simulink model "step3c"  (Simulink 8.5)
settings: Solver=ode15s  SolverMode=SingleTasking  StartTime=0.0  StopTime=0.199  RelTol=1e-4  AbsTol=1e-6
undefined symbols (not defined in the file or in its folder): den, dx, num
libraries: elements x1
settings Model: Creator=PC  LastModifiedBy=PC
settings DataIOCC: LimitDataPoints=off
settings OptimizationCC: BlockReduction=off  BooleanDataType=off  ExpressionDepthLimit=128
settings DebuggingCC: SaveWithParameterizedLinksMsg=none  SignalResolutionControl=TryResolveAllWithWarning  MultiTaskDSMMsg=warning  MultiTaskCondExecSysMsg=none  FcnCallInpInsideContextMsg=EnableAllAsError  StateNameClashWarn=none  StrictBusMsg=None
settings HardwareCC: TargetUnknown=on
settings RTWCC: TemplateMakefile=grt_vc.tmf

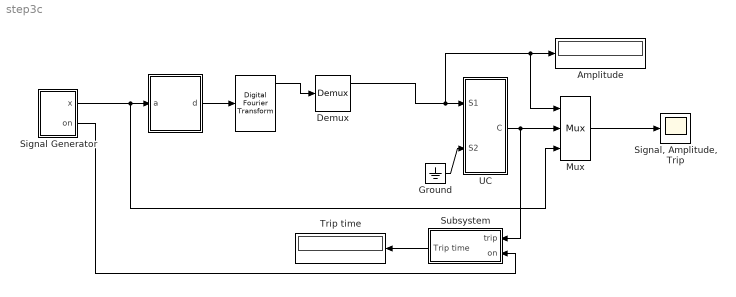
== system step3c ==
  " " : elements/   fo=60  window_size=20  harmonic=[1 2 3 4 5]
  "  " : Subsystem  mask(Data Adquisition Board){filter=on, approx=Butterworth, order=3, numerator=[], denominator=[], freq=180, resdis=on, vertres=8, xmax=100, winsize=20, G=1.0, fs=60*20}
      mask prompts: filter "Disable Analog Filter"; approx "Filter approximation"; numerator "Free expression filter: numerator(descending order of s)"; denominator "Free expression filter: denominator:"; freq "Cut-off frequency"; resdis "Disable Vertical Resolution"; vertres "Vertical Resolution: No. of bits"; xmax "Vertical Resolution: signal range"; winsize "Window size"; G "Gain"; fs "Sampling frequency"
      mask help: Takes the instantaneous value of the input signal and convert it to the data window of samples.
      mask init:
      | dab1
      mask TypeOptions approx: Bessel | Tschebyscheff | Butterworth | free expression
      mask TypeOptions order: 2 | 3 | 4
      mask TypeOptions vertres: 8 | 12 | 16
      mask Display: disp('DAB')
  Amplitude : Display
  Demux : Demux  Outputs=2
  Ground : Ground
  Mux : Mux  Inputs=3
  Signal Generator : Subsystem  mask(Signal Generator){A1=2, f1=60, A2=0, f2=2*60, A3=0, f3=1500, tstart=1.25/60}
      mask prompts: A1 "Amplitude 1"; f1 "Frequency 1 [Hz]"; A2 "Amplitude 2"; f2 "Frequency 2 [Hz]"; A3 "Amplitude 3"; f3 "Frequency 3 [Hz]"; tstart "Start time [sec]"
  "Signal, Amplitude, Trip" : Scope
      settings: TickLabels=on  YMin=-4.5  YMax=4.5
  Subsystem : Subsystem
  Trip time : Display
  UC : Subsystem  mask(Universal Comparator){type2=Signal-Time, sign=>, Ipickup=0.75, k1=0.95, type1=Very Inverse, type3=Present value, k=0.015, fs=20*60}
      mask prompts: type2 "Type of comparison"; Ipickup "Pick-up value:"; k1 "Ratio of reset to pick-up:"; type1 "Type of Time dependency"; type3 "I-t emulation method"; k "Time parameter (seconds):"; fs "Sampling frecuency (Hz):"
      mask help: This block is an Universal Comparator. It can perform a comparison between a signal an a threshold or two signals. It can also emulate some time-signal characteristics.
      mask init:
      | switch type2,
      |    case 1,
      |        %signal-threshold
      |        if sign ==1
      |           %S1>S2
      |           aux=0;
      |        else
      |           %S1<S2
      |           aux=1;
      |        end;
      |    case 2,
      |        %Signal-Signal
      |       if sign ==1
      |           aux=2;
      |    	else
      |          aux=3;
      |       end;
      |    case 3,
      |       %signal-time
      |       if type3==1
      |          %instantaneous value of input signal
      |          switch type1,
      |             case 1,
      |                %time defined
      |                aux=4;
      |             case 2,
      |                %inverse time
      |                aux=6;
      |             case 3,
      |                %very inverse
      |                aux=7;
      |             case 4,
      |                %extremely inverse
      |                aux=8;
      |             case 5,
      |                %RI inverse
      |                aux=9;
      |             case 6,
      |                %Long time inverse
      |                aux=10;
      |             otherwise,
      |                aux=0;
      |          end;
      |       else
      |          switch type1,
      |             case 1,
      |                %time defined
      |                aux=5;
      |             case 2,
      |                %inverse time
      |                aux=11;
      |             case 3,
      |                %very inverse
      |                aux=12;
      |             case 4,
      |                %extremely inverse
      |                aux=13;
      |             case 5,
      |                %RI inverse
      |                aux=14;
      |             case 6,
      |                %Long time inverse
      |                aux=15;
      |             otherwise,
      |                aux=0;
      |          end;
      |       end;
      |    otherwise,
      |          aux=0;
      | end;
      mask TypeOptions type2: Signal-Threshold | Signal-Signal | Signal-Time
      mask TypeOptions sign: > | <
      mask TypeOptions type1: Time defined | Standard Inverse | Very Inverse | Extra Inverse | RI Inverse | Long Time Inverse
      mask TypeOptions type3: Present value | integration
      mask Display: disp('UC');
  wires:
  Signal Generator/1(x) -> "  "/1(a), Mux/3
  "  "/1(d) -> " "/1
  " "/1 -> Demux/1
  Signal Generator/2(on) -> Subsystem/2(on)
  Subsystem/1(Trip time) -> Trip time/1
  UC/1(C) -> Subsystem/1(trip), Mux/2
  Mux/1 -> "Signal, Amplitude, Trip"/1
  Ground/1 -> UC/2(S2)
  Demux/1 -> UC/1(S1), Amplitude/1, Mux/1

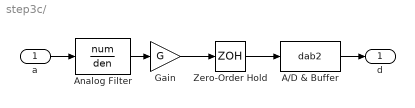
== system step3c/   ==
  a : Inport
  A/D & Buffer : S-Function  FunctionName=dab2  Parameters=winsize,fs,dx,resdis
  Analog Filter : TransferFcn  Numerator=num  Denominator=den
  Gain : Gain  Gain=G  SaturateOnIntegerOverflow=on  OutDataTypeStr=Inherit: Same as input  ParamDataTypeStr=Inherit: Same as input
  Zero-Order Hold : ZeroOrderHold  SampleTime=1/fs
  d : Outport  InitialOutput=[zeros(winsize,1)]
  wires:
  A/D & Buffer/1 -> d/1
  a/1 -> Analog Filter/1
  Zero-Order Hold/1 -> A/D & Buffer/1
  Gain/1 -> Zero-Order Hold/1
  Analog Filter/1 -> Gain/1

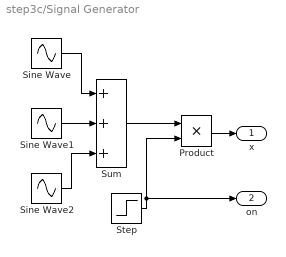
== system step3c/Signal Generator ==
  Product : Product  SaturateOnIntegerOverflow=on  RndMeth=Zero  InputSameDT=on  OutDataTypeStr=Inherit: Same as first input
  Sine Wave : Sin  Amplitude=A1  Frequency=f1*2*pi  SampleTime=0
  Sine Wave1 : Sin  Amplitude=A2  Frequency=f2*2*pi  SampleTime=0
  Sine Wave2 : Sin  Amplitude=A3  Frequency=f3*2*pi  SampleTime=0
  Step : Step  Time=tstart
  Sum : Sum  Inputs=+++  SaturateOnIntegerOverflow=on  InputSameDT=on  OutDataTypeStr=Inherit: Same as first input
  x : Outport  InitialOutput=0
  on : Outport  Port=2  InitialOutput=0
  wires:
  Step/1 -> on/1, Product/2
  Product/1 -> x/1
  Sum/1 -> Product/1
  Sine Wave2/1 -> Sum/3
  Sine Wave1/1 -> Sum/2
  Sine Wave/1 -> Sum/1

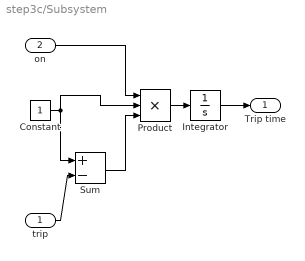
== system step3c/Subsystem ==
  trip : Inport
  on : Inport  Port=2
  Constant : Constant
  Integrator : Integrator
  Product : Product  Inputs=3  SaturateOnIntegerOverflow=on  RndMeth=Zero  InputSameDT=on  OutDataTypeStr=Inherit: Same as first input
  Sum : Sum  Inputs=+-  SaturateOnIntegerOverflow=on  InputSameDT=on  OutDataTypeStr=Inherit: Same as first input
  Trip time : Outport  InitialOutput=0
  wires:
  on/1 -> Product/1
  Sum/1 -> Product/3
  Integrator/1 -> Trip time/1
  Product/1 -> Integrator/1
  Constant/1 -> Sum/1, Product/2
  trip/1 -> Sum/2

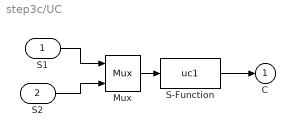
== system step3c/UC ==
  S1 : Inport
  S2 : Inport  Port=2
  Mux : Mux  Inputs=2
  S-Function : S-Function  FunctionName=uc1  Parameters=k,k1,aux,Ipickup,fs
  C : Outport  InitialOutput=0
  wires:
  S-Function/1 -> C/1
  Mux/1 -> S-Function/1
  S1/1 -> Mux/1
  S2/1 -> Mux/2
